simulink model "modelo"  (R2016b)
settings: Solver=VariableStepAuto  StartTime=0.0  StopTime=100.0  FixedStep=0.00001  RelTol=1e-3
values from neighbouring files (symbols this model uses):
  K = 0.36783    [carregaDados.m]    (also in carregaDadosDoModelo.m = 0.01332; carregaDadosSimulacao.m = 0.01)
  tau = 13.314    [carregaDados.m]    (also in carregaDadosSimulacao.m)
settings Model: Creator=maripimentel  LastModifiedBy=maripimentel

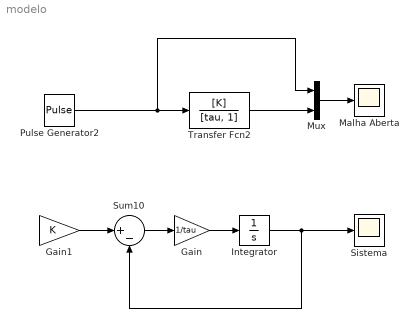
== system modelo ==
  Gain : Gain  Gain=1/tau
  Gain1 : Gain  Gain=K
  Integrator : Integrator
  "Malha Aberta " : Scope
  Mux : Mux  Inputs=2
  Pulse Generator2 : DiscretePulseGenerator  PulseType=Time based  Period=1000  PulseWidth=50
  "Sistema " : Scope
  Sum10 : Sum  Inputs=|+-
  Transfer Fcn2 : TransferFcn  Numerator=[K]  Denominator=[tau, 1]
  wires:
  Sum10/1 -> Gain/1
  Integrator/1 -> Sum10/2, "Sistema "/1
  Gain1/1 -> Sum10/1
  Gain/1 -> Integrator/1
  Mux/1 -> "Malha Aberta "/1
  Pulse Generator2/1 -> Mux/1, Transfer Fcn2/1
  Transfer Fcn2/1 -> Mux/2
